simulink model "g"  (R2021a)
settings: Solver=VariableStepAuto  StartTime=0.0  StopTime=10.0  RelTol=1e-3
settings Model: Creator=Ajay M  LastModifiedBy=Ajay M

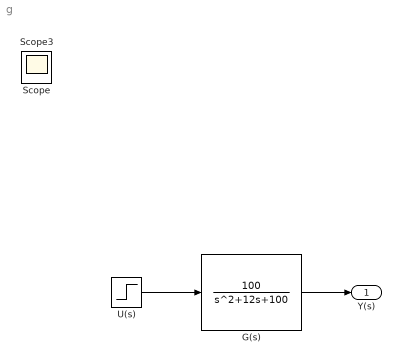
== system g ==
  G(s) : TransferFcn  Numerator=[100]  Denominator=[1 12 100]
  U(s) : Step  SampleTime=0
  Y(s) : Outport
  Scope : Scope
  Scope3 : Scope
  wires:
  G(s)/1 -> Y(s)/1
  U(s)/1 -> G(s)/1
